simulink model "PARACHUTE"  (R2022b)
settings: Solver=VariableStepAuto  StartTime=0.0  StopTime=10.0  RelTol=1e-3
settings Model: Creator=lucaerviati  LastModifiedBy=lucaerviati

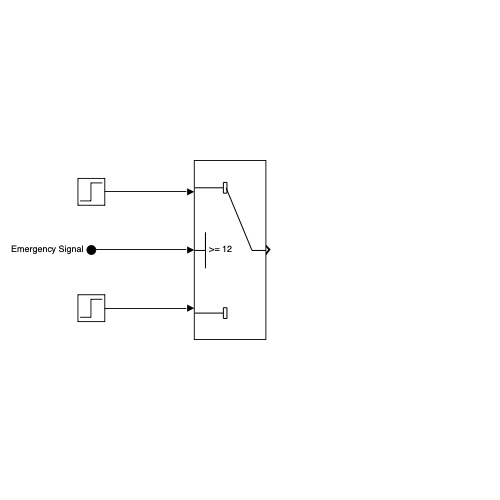
[thumbnail: Simulink's stored preview of the top-level diagram]
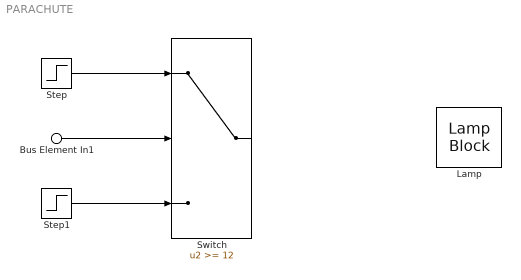
== system PARACHUTE ==
  Bus Element In1 : Inport  PortName=Emergency Signal
  Lamp : LampBlock  LabelPosition=Hide  Icon=Ex1
  Step : Step  After=12  SampleTime=0
  Step1 : Step  After=0  SampleTime=0
  Switch : Switch  Threshold=12  SaturateOnIntegerOverflow=off  InputSameDT=off
  wires:
  Bus Element In1/1 -> Switch/2
  Step/1 -> Switch/1
  Step1/1 -> Switch/3
